simulink model "hw2a"  (R2017a)
settings: Solver=VariableStepAuto  StartTime=0.0  StopTime=10.0  RelTol=1e-3
settings Model: Creator=Soutrik  LastModifiedBy=Soutrik

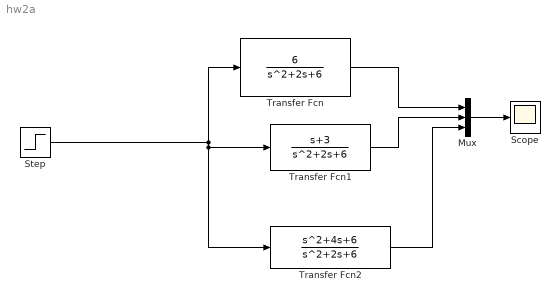
== system hw2a ==
  Mux : Mux  Inputs=3
  Scope : Scope
  Step : Step  SampleTime=0
  Transfer Fcn : TransferFcn  Numerator=[6]  Denominator=[1 2 6]
  Transfer Fcn1 : TransferFcn  Numerator=[1 3]  Denominator=[1 2 6]
  Transfer Fcn2 : TransferFcn  Numerator=[1 4 6]  Denominator=[1 2 6]
  wires:
  Step/1 -> Transfer Fcn2/1, Transfer Fcn1/1, Transfer Fcn/1
  Transfer Fcn/1 -> Mux/1
  Transfer Fcn1/1 -> Mux/2
  Transfer Fcn2/1 -> Mux/3
  Mux/1 -> Scope/1
